simulink model "observer_model_dist"  (R2018b)
settings: Solver=VariableStepAuto  StartTime=0.0  StopTime=0.5  RelTol=1e-3
values from neighbouring files (symbols this model uses):
  K = 20    [continous_controller.m]    (also in control_input_bound.m = place(sys_discrete.A, sys_discrete.B, discrete_poles); delayed_input.m = place(sys_discrete.A, sys_discrete.B, discrete_poles); discrete_pole_placement.m = place(sys_discrete.A, sys_discrete.B, discrete_poles); pole_placement_delay.m = place(sys.A, sys.B, continous_poles))
  K_obs = K_obs'    [discrete_pole_placement.m]
  k_r = k_r(1)^-1    [discrete_pole_placement.m]    (also in lqr_delay.m = 30)
  sys_discrete = c2d(sys, 2*pi/sampling_freq, 'zoh')    [control_input_bound.m]    (also in delayed_input.m = (c2d(sys, 2*pi/sampling_freq, 'zoh')); discrete_pole_placement.m = (c2d(sys, 2*pi/sampling_freq, 'zoh')); discretization.m; lqr_controller.m)
undefined symbols (not defined in the file or in its folder): DiscIntNeverNeededParam
settings Model: Creator=lorenzoterenzi  LastModifiedBy=lorenzoterenzi

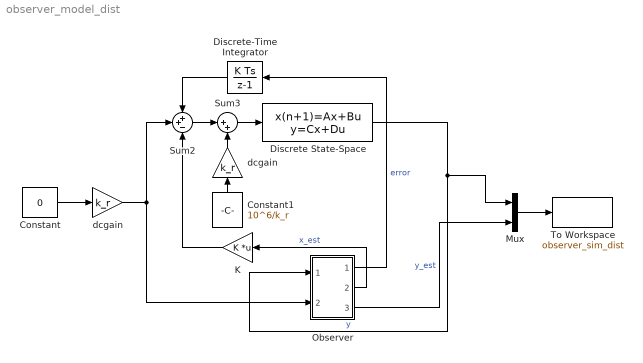
== system observer_model_dist ==
  Constant : Constant  Value=0
  Constant1 : Constant  Value=10^6/k_r
  Discrete State-Space : DiscreteStateSpace  A=sys_discrete.A  B=sys_discrete.B  C=sys_discrete.C  D=sys_discrete.D  InitialCondition=[0, 0, 0, 0];  SampleTime=sys_discrete.Ts
  Discrete-Time Integrator : DiscreteIntegrator  gainval=10^10  SampleTime=sys_discrete.Ts  ICPrevOutput=DiscIntNeverNeededParam  ICPrevScaledInput=DiscIntNeverNeededParam
  K : Gain  Gain=K  Multiplication=Matrix(K*u)
  Mux : Mux  Inputs=2
  Observer : Subsystem
  Sum2 : Sum  Inputs=++-
  Sum3 : Sum  Inputs=|++
  To Workspace : ToWorkspace  VariableName=observer_sim_dist  SaveFormat=Timeseries  SampleTime=-1
  dcgain : Gain  Gain=k_r
  "dcgain " : Gain  Gain=k_r
  wires:
  Constant/1 -> "dcgain "/1
  Mux/1 -> To Workspace/1
  "dcgain "/1 -> Observer/2(In2), Sum2/2
  Sum2/1 -> Sum3/1
  Sum3/1 -> Discrete State-Space/1
  Constant1/1 -> dcgain/1
  Discrete State-Space/1 -> Observer/1(In1), Mux/1  "y"
  K/1 -> Sum2/3
  Discrete-Time Integrator/1 -> Sum2/1
  Observer/1(Out1) -> Discrete-Time Integrator/1  "error"
  Observer/2(Out2) -> K/1  "x_est"
  Observer/3(Out3) -> Mux/2  "y_est"
  dcgain/1 -> Sum3/2

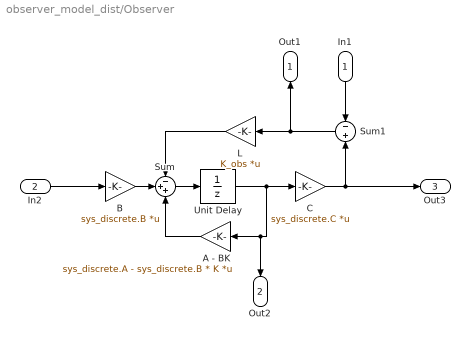
== system observer_model_dist/Observer ==
  In1 : Inport
  In2 : Inport  Port=2
  A - BK : Gain  Gain=sys_discrete.A - sys_discrete.B * K  Multiplication=Matrix(K*u)
  B : Gain  Gain=sys_discrete.B  Multiplication=Matrix(K*u)
  C : Gain  Gain=sys_discrete.C  Multiplication=Matrix(K*u)
  L : Gain  Gain=K_obs  Multiplication=Matrix(K*u)
  Sum : Sum  Inputs=-++
  Sum1 : Sum  Inputs=-|+
  Unit Delay : UnitDelay  SampleTime=sys_discrete.Ts
  Out1 : Outport
  Out2 : Outport  Port=2
  Out3 : Outport  Port=3
  wires:
  L/1 -> Sum/1
  Sum/1 -> Unit Delay/1
  In2/1 -> B/1
  Unit Delay/1 -> A - BK/1, Out2/1, C/1
  Sum1/1 -> L/1, Out1/1
  C/1 -> Out3/1, Sum1/2
  In1/1 -> Sum1/1
  A - BK/1 -> Sum/3
  B/1 -> Sum/2
